simulink model "Eskf"  (R2025b)
settings: Solver=FixedStepDiscrete  StartTime=0.0  StopTime=100  FixedStep=Ts_10us  RelTol=1e-3
model workspace (MAT data in the model file):
  B_const = Simulink.Parameter
  B_const.Value = [1; 0; 0]
  B_const.Complexity = 'real'
  B_const.Dimensions = [3 1]
  B_const.DataType = 'auto'
  Param = Simulink.Parameter
  Param.Complexity = 'real'
  Param.Dimensions = [0 0]
  Param.DataType = 'auto'
  Ts_100us = Simulink.Parameter
  Ts_100us.Value = 0.0001
  Ts_100us.Complexity = 'real'
  Ts_100us.Dimensions = [1 1]
  Ts_100us.DataType = 'auto'
  Ts_10us = Simulink.Parameter
  Ts_10us.Value = 1e-05
  Ts_10us.Complexity = 'real'
  Ts_10us.Dimensions = [1 1]
  Ts_10us.DataType = 'auto'
  Ts_acc = Simulink.Parameter
  Ts_acc.Value = 0.0001
  Ts_acc.Complexity = 'real'
  Ts_acc.Dimensions = [1 1]
  Ts_acc.DataType = 'auto'
  Ts_eskf = Simulink.Parameter
  Ts_eskf.Value = 0.0001
  Ts_eskf.Complexity = 'real'
  Ts_eskf.Dimensions = [1 1]
  Ts_eskf.DataType = 'auto'
  Ts_gps = Simulink.Parameter
  Ts_gps.Value = 0.0001
  Ts_gps.Complexity = 'real'
  Ts_gps.Dimensions = [1 1]
  Ts_gps.DataType = 'auto'
  Ts_gyro = Simulink.Parameter
  Ts_gyro.Value = 0.0001
  Ts_gyro.Complexity = 'real'
  Ts_gyro.Dimensions = [1 1]
  Ts_gyro.DataType = 'auto'
  Ts_mag = Simulink.Parameter
  Ts_mag.Value = 0.0001
  Ts_mag.Complexity = 'real'
  Ts_mag.Dimensions = [1 1]
  Ts_mag.DataType = 'auto'
  acc_bias_static = Simulink.Parameter
  acc_bias_static.Value = [0.01; -0.01; 0.01]
  acc_bias_static.Complexity = 'real'
  acc_bias_static.Dimensions = [3 1]
  acc_bias_static.DataType = 'auto'
  g = Simulink.Parameter
  g.Value = [0; 0; 9.80665]
  g.Complexity = 'real'
  g.Dimensions = [3 1]
  g.DataType = 'auto'
  omega_bias_static = Simulink.Parameter
  omega_bias_static.Value = [0.01; -0.01; 0.01]
  omega_bias_static.Complexity = 'real'
  omega_bias_static.Dimensions = [3 1]
  omega_bias_static.DataType = 'auto'
  var_B_n = Simulink.Parameter
  var_B_n.Value = Simulink.data.Expression
  var_B_n.Value.ExpressionString = "0.001*[0.001;0.001;0.001]"
  var_B_n.Complexity = 'real'
  var_B_n.Dimensions = -1
  var_B_n.DataType = 'auto'
  var_a_n = Simulink.Parameter
  var_a_n.Value = Simulink.data.Expression
  var_a_n.Value.ExpressionString = "0.001"
  var_a_n.Complexity = 'real'
  var_a_n.Dimensions = -1
  var_a_n.DataType = 'auto'
  var_a_w = Simulink.Parameter
  var_a_w.Value = Simulink.data.Expression
  var_a_w.Value.ExpressionString = "0.001"
  var_a_w.Complexity = 'real'
  var_a_w.Dimensions = -1
  var_a_w.DataType = 'auto'
  var_pos_n = Simulink.Parameter
  var_pos_n.Value = Simulink.data.Expression
  var_pos_n.Value.ExpressionString = "0.001*[1;1;1]"
  var_pos_n.Complexity = 'real'
  var_pos_n.Dimensions = -1
  var_pos_n.DataType = 'auto'
  var_vel_n = Simulink.Parameter
  var_vel_n.Value = Simulink.data.Expression
  var_vel_n.Value.ExpressionString = "0.001*[0.1;0.1;0.1]"
  var_vel_n.Complexity = 'real'
  var_vel_n.Dimensions = -1
  var_vel_n.DataType = 'auto'
  var_w_n = Simulink.Parameter
  var_w_n.Value = Simulink.data.Expression
  var_w_n.Value.ExpressionString = "0.001"
  var_w_n.Complexity = 'real'
  var_w_n.Dimensions = -1
  var_w_n.DataType = 'auto'
  var_w_w = Simulink.Parameter
  var_w_w.Value = Simulink.data.Expression
  var_w_w.Value.ExpressionString = "0.001"
  var_w_w.Complexity = 'real'
  var_w_w.Dimensions = -1
  var_w_w.DataType = 'auto'
undefined symbols (not defined in the file): DiscIntNeverNeededParam
libraries: simulink x4
settings Model: Creator=unimage  LastModifiedBy=unimage
settings DebuggingCC: SignalInfNanChecking=error  CheckMatrixSingularityMsg=error

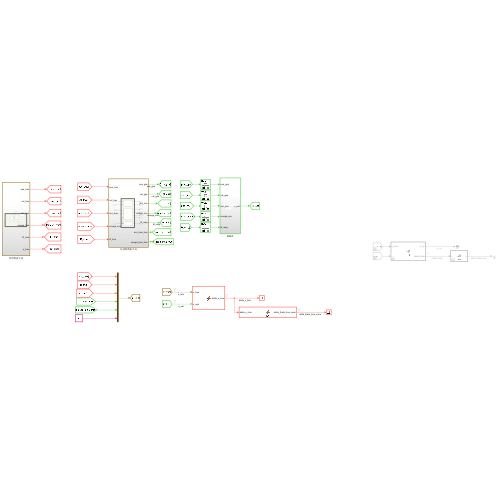
[thumbnail: Simulink's stored preview of the top-level diagram]
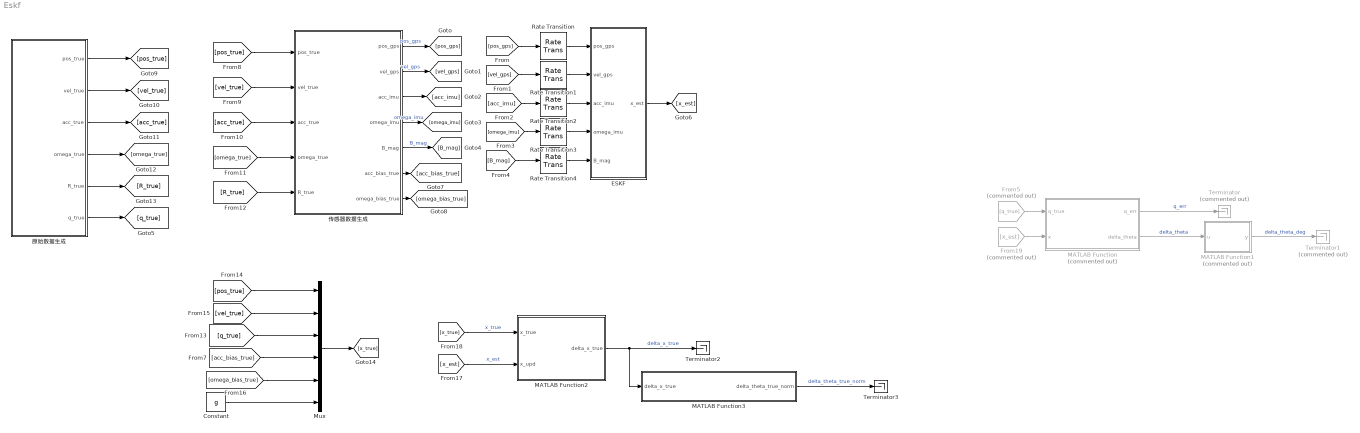
== system Eskf ==
  Constant : Constant  Value=g
  ESKF : Subsystem
  From19 : From  Commented=on  GotoTag=x_est
  From5 : From  Commented=on  GotoTag=q_true
  MATLAB Function : MATLAB Function  Commented=on  TreatAsAtomicUnit=on
  MATLAB Function1 : MATLAB Function  Commented=on  TreatAsAtomicUnit=on
  MATLAB Function2 : MATLAB Function  TreatAsAtomicUnit=on
  MATLAB Function3 : MATLAB Function  TreatAsAtomicUnit=on
  Mux : Mux  Inputs=6
  Rate Transition{,1..4} (5 alike) : RateTransition  OutPortSampleTime=Ts_eskf
  Terminator : Terminator  Commented=on
  Terminator1 : Terminator  Commented=on
  Terminator2 : Terminator
  Terminator3 : Terminator
  传感器数据生成 : Subsystem
  原始数据生成 : Subsystem
  wires:
  传感器数据生成/1(pos_gps) -> [pos_gps]  "pos_gps"
  传感器数据生成/2(vel_gps) -> [vel_gps]  "vel_gps"
  传感器数据生成/3(acc_imu) -> [acc_imu]
  传感器数据生成/4(omega_imu) -> [omega_imu]  "omega_imu"
  传感器数据生成/5(B_mag) -> [B_mag]  "B_mag"
  [pos_gps] -> Rate Transition/1
  [vel_gps] -> Rate Transition1/1
  [acc_imu] -> Rate Transition2/1
  [omega_imu] -> Rate Transition3/1
  [B_mag] -> Rate Transition4/1
  Rate Transition/1 -> ESKF/1(pos_gps)
  Rate Transition1/1 -> ESKF/2(vel_gps)
  Rate Transition2/1 -> ESKF/3(acc_imu)
  Rate Transition3/1 -> ESKF/4(omega_imu)
  Rate Transition4/1 -> ESKF/5(B_mag)
  原始数据生成/6(q_true) -> [q_true]
  ESKF/1(x_est) -> [x_est]
  From5/1 -> MATLAB Function/1(q_true)
  From19/1 -> MATLAB Function/2(x)
  MATLAB Function/1(q_err) -> Terminator/1  "q_err"
  MATLAB Function/2(delta_theta) -> MATLAB Function1/1(u)  "delta_theta"
  MATLAB Function1/1(y) -> Terminator1/1  "delta_theta_deg"
  传感器数据生成/6(acc_bias_true) -> [acc_bias_true]
  传感器数据生成/7(omega_bias_true) -> [omega_bias_true]
  原始数据生成/1(pos_true) -> [pos_true]
  原始数据生成/3(acc_true) -> [acc_true]
  原始数据生成/2(vel_true) -> [vel_true]
  原始数据生成/4(omega_true) -> [omega_true]
  原始数据生成/5(R_true) -> [R_true]
  [pos_true] -> 传感器数据生成/1(pos_true)
  [vel_true] -> 传感器数据生成/2(vel_true)
  [acc_true] -> 传感器数据生成/3(acc_true)
  [omega_true] -> 传感器数据生成/4(omega_true)
  [R_true] -> 传感器数据生成/5(R_true)
  [acc_bias_true] -> Mux/4
  [q_true] -> Mux/3
  [pos_true] -> Mux/1
  [vel_true] -> Mux/2
  [omega_bias_true] -> Mux/5
  Constant/1 -> Mux/6
  Mux/1 -> [x_true]
  [x_true] -> MATLAB Function2/1(x_true)  "x_true"
  [x_est] -> MATLAB Function2/2(x_upd)  "x_est"
  MATLAB Function2/1(delta_x_true) -> MATLAB Function3/1(delta_x_true), Terminator2/1  "delta_x_true"
  MATLAB Function3/1(delta_theta_true_norm) -> Terminator3/1  "delta_theta_true_norm"

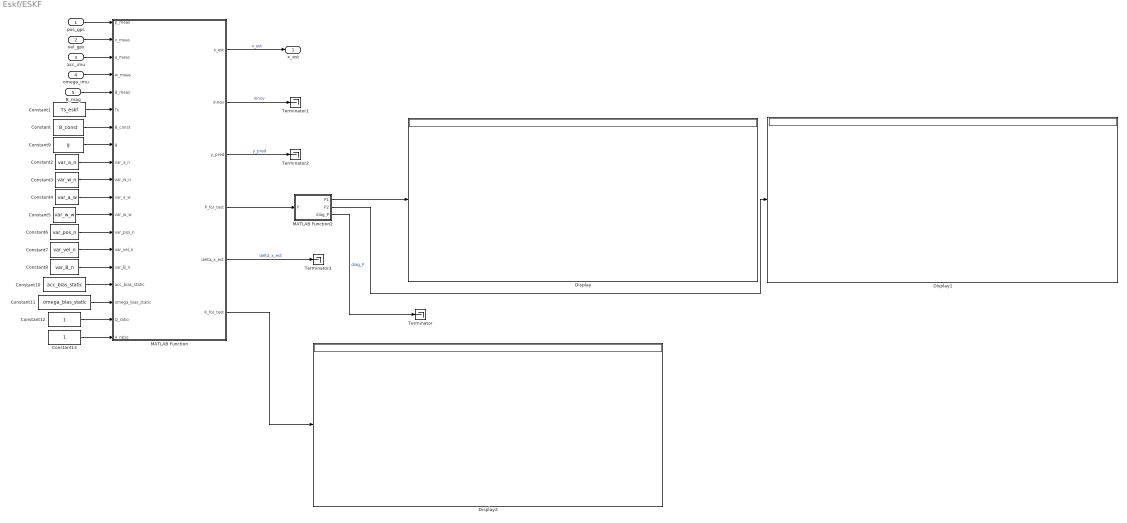
== system Eskf/ESKF ==
  pos_gps : Inport
  vel_gps : Inport  Port=2
  acc_imu : Inport  Port=3
  omega_imu : Inport  Port=4
  B_mag : Inport  Port=5
  Constant : Constant  Value=B_const
  Constant1 : Constant  Value=Ts_eskf
  Constant10 : Constant  Value=acc_bias_static
  Constant11 : Constant  Value=omega_bias_static
  Constant12 : Constant
  Constant13 : Constant
  Constant2 : Constant  Value=var_a_n
  Constant3 : Constant  Value=var_w_n
  Constant4 : Constant  Value=var_a_w
  Constant5 : Constant  Value=var_w_w
  Constant6 : Constant  Value=var_pos_n
  Constant7 : Constant  Value=var_vel_n
  Constant8 : Constant  Value=var_B_n
  Constant9 : Constant  Value=g
  Display : Display
      settings: Format=bank
  Display1 : Display
      settings: Format=bank
  Display2 : Display
      settings: Format=bank
  MATLAB Function : MATLAB Function  TreatAsAtomicUnit=on
  MATLAB Function2 : MATLAB Function  TreatAsAtomicUnit=on
  Terminator{,1..3} (4 alike) : Terminator
  x_est : Outport
  wires:
  pos_gps/1 -> MATLAB Function/1(p_meas)
  vel_gps/1 -> MATLAB Function/2(v_meas)
  acc_imu/1 -> MATLAB Function/3(a_meas)
  omega_imu/1 -> MATLAB Function/4(w_meas)
  B_mag/1 -> MATLAB Function/5(B_meas)
  Constant1/1 -> MATLAB Function/6(Ts)
  Constant/1 -> MATLAB Function/7(B_const)
  Constant2/1 -> MATLAB Function/9(var_a_n)
  Constant3/1 -> MATLAB Function/10(var_w_n)
  Constant4/1 -> MATLAB Function/11(var_a_w)
  Constant5/1 -> MATLAB Function/12(var_w_w)
  MATLAB Function/1(x_est) -> x_est/1  "x_est"
  MATLAB Function/2(innov) -> Terminator1/1  "innov"
  Constant6/1 -> MATLAB Function/13(var_pos_n)
  Constant7/1 -> MATLAB Function/14(var_vel_n)
  Constant8/1 -> MATLAB Function/15(var_B_n)
  MATLAB Function/3(y_pred) -> Terminator2/1  "y_pred"
  MATLAB Function/4(P_for_test) -> MATLAB Function2/1(P)
  MATLAB Function2/1(P1) -> Display/1
  MATLAB Function2/2(P2) -> Display1/1
  MATLAB Function2/3(diag_P) -> Terminator/1  "diag_P"
  MATLAB Function/5(delta_x_est) -> Terminator3/1  "delta_x_est"
  Constant9/1 -> MATLAB Function/8(g)
  Constant10/1 -> MATLAB Function/16(acc_bias_static)
  Constant11/1 -> MATLAB Function/17(omega_bias_static)
  Constant12/1 -> MATLAB Function/18(Q_ratio)
  Constant13/1 -> MATLAB Function/19(V_ratio)
  MATLAB Function/6(K_for_test) -> Display2/1

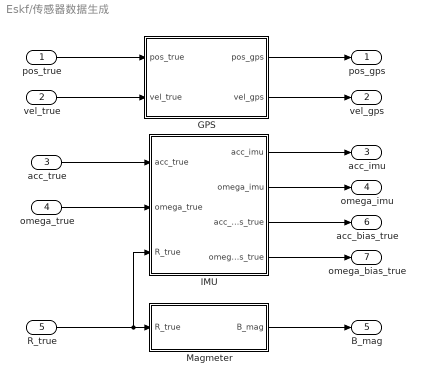
== system Eskf/传感器数据生成 ==
  pos_true : Inport
  vel_true : Inport  Port=2
  acc_true : Inport  Port=3
  omega_true : Inport  Port=4
  R_true : Inport  Port=5
  GPS : Subsystem
  IMU : Subsystem
  Magmeter : Subsystem
  pos_gps : Outport
  vel_gps : Outport  Port=2
  acc_imu : Outport  Port=3
  omega_imu : Outport  Port=4
  B_mag : Outport  Port=5
  acc_bias_true : Outport  Port=6
  omega_bias_true : Outport  Port=7
  wires:
  vel_true/1 -> GPS/2(vel_true)
  R_true/1 -> IMU/3(R_true), Magmeter/1(R_true)
  omega_true/1 -> IMU/2(omega_true)
  IMU/2(omega_imu) -> omega_imu/1
  IMU/1(acc_imu) -> acc_imu/1
  Magmeter/1(B_mag) -> B_mag/1
  acc_true/1 -> IMU/1(acc_true)
  pos_true/1 -> GPS/1(pos_true)
  GPS/1(pos_gps) -> pos_gps/1
  GPS/2(vel_gps) -> vel_gps/1
  IMU/3(acc_bias_true) -> acc_bias_true/1
  IMU/4(omega_bias_true) -> omega_bias_true/1

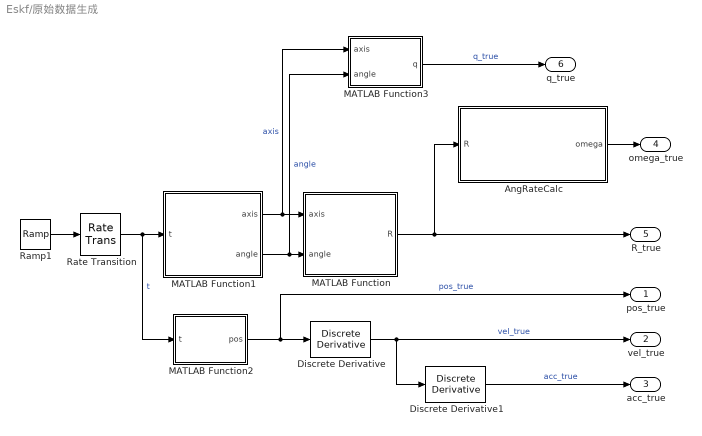
== system Eskf/原始数据生成 ==
  AngRateCalc : Subsystem
  Discrete Derivative : simulink/Discrete/Discrete Derivative  gainval=1.0  ICPrevScaledInput=0.0  OutMin=[]  OutMax=[]  OutDataType=fixdt(1, 16)  OutScaling=2^-10  DoSatur=off
  Discrete Derivative1 : simulink/Discrete/Discrete Derivative  gainval=1.0  ICPrevScaledInput=0.0  OutMin=[]  OutMax=[]  OutDataType=fixdt(1, 16)  OutScaling=2^-10  DoSatur=off
  MATLAB Function : MATLAB Function  TreatAsAtomicUnit=on
  MATLAB Function1 : MATLAB Function  TreatAsAtomicUnit=on
  MATLAB Function2 : MATLAB Function  TreatAsAtomicUnit=on
  MATLAB Function3 : MATLAB Function  TreatAsAtomicUnit=on
  Ramp1 : simulink/Sources/Ramp  slope=1  start=0  InitialOutput=0
  Rate Transition : RateTransition  OutPortSampleTime=Ts_10us
  pos_true : Outport
  vel_true : Outport  Port=2
  acc_true : Outport  Port=3
  omega_true : Outport  Port=4
  R_true : Outport  Port=5
  q_true : Outport  Port=6
  wires:
  MATLAB Function1/1(axis) -> MATLAB Function3/1(axis), MATLAB Function/1(axis)  "axis"
  MATLAB Function1/2(angle) -> MATLAB Function3/2(angle), MATLAB Function/2(angle)  "angle"
  MATLAB Function2/1(pos) -> pos_true/1, Discrete Derivative/1  "pos_true"
  Ramp1/1 -> Rate Transition/1
  Rate Transition/1 -> MATLAB Function2/1(t), MATLAB Function1/1(t)  "t"
  Discrete Derivative/1 -> vel_true/1, Discrete Derivative1/1  "vel_true"
  Discrete Derivative1/1 -> acc_true/1  "acc_true"
  AngRateCalc/1(omega) -> omega_true/1
  MATLAB Function/1(R) -> AngRateCalc/1(R), R_true/1
  MATLAB Function3/1(q) -> q_true/1  "q_true"

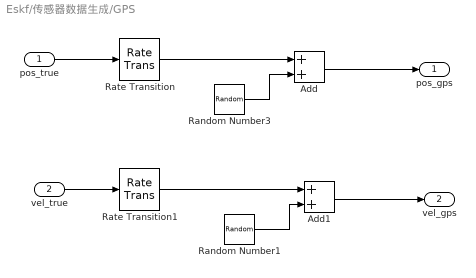
== system Eskf/传感器数据生成/GPS ==
  pos_true : Inport
  vel_true : Inport  Port=2
  Add : Sum
  Add1 : Sum
  Random Number1 : RandomNumber  Mean=[0 0 0]  Variance=var_vel_n  Seed=[0 1 2]  SampleTime=Ts_gps
  Random Number3 : RandomNumber  Mean=[0 0 0]  Variance=var_pos_n  Seed=[0 1 2]  SampleTime=Ts_gps
  Rate Transition : RateTransition  OutPortSampleTime=Ts_gps
  Rate Transition1 : RateTransition  OutPortSampleTime=Ts_gps
  pos_gps : Outport
  vel_gps : Outport  Port=2
  wires:
  pos_true/1 -> Rate Transition/1
  Random Number3/1 -> Add/2
  Add/1 -> pos_gps/1
  Random Number1/1 -> Add1/2
  vel_true/1 -> Rate Transition1/1
  Add1/1 -> vel_gps/1
  Rate Transition/1 -> Add/1
  Rate Transition1/1 -> Add1/1

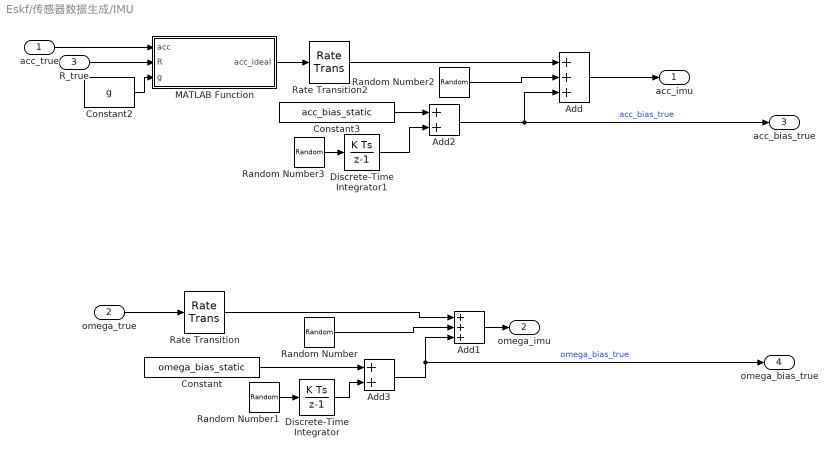
== system Eskf/传感器数据生成/IMU ==
  acc_true : Inport
  omega_true : Inport  Port=2
  R_true : Inport  Port=3
  Add : Sum  Inputs=+++
  Add1 : Sum  Inputs=+++
  Add2 : Sum
  Add3 : Sum
  Constant : Constant  Value=omega_bias_static
  Constant2 : Constant  Value=g
  Constant3 : Constant  Value=acc_bias_static
  Discrete-Time Integrator : DiscreteIntegrator  SampleTime=-1  ICPrevOutput=DiscIntNeverNeededParam  ICPrevScaledInput=DiscIntNeverNeededParam
  Discrete-Time Integrator1 : DiscreteIntegrator  SampleTime=-1  ICPrevOutput=DiscIntNeverNeededParam  ICPrevScaledInput=DiscIntNeverNeededParam
  MATLAB Function : MATLAB Function  TreatAsAtomicUnit=on
  Random Number : RandomNumber  Mean=[0 0 0]  Variance=var_w_n*ones(3,1)  Seed=[0 1 2]  SampleTime=Ts_gyro
  Random Number1 : RandomNumber  Mean=[0 0 0]  Variance=var_w_w*ones(3,1)  Seed=[3 4 5]  SampleTime=Ts_gyro
  Random Number2 : RandomNumber  Mean=[0 0 0]  Variance=var_a_n*ones(3,1)  Seed=[9 10 11]  SampleTime=Ts_acc
  Random Number3 : RandomNumber  Mean=[0 0 0]  Variance=var_a_w*ones(3,1)  Seed=[6 7 8]  SampleTime=Ts_acc
  Rate Transition : RateTransition  OutPortSampleTime=Ts_gyro
  Rate Transition2 : RateTransition  OutPortSampleTime=Ts_acc
  acc_imu : Outport
  omega_imu : Outport  Port=2
  acc_bias_true : Outport  Port=3
  omega_bias_true : Outport  Port=4
  wires:
  acc_true/1 -> MATLAB Function/1(acc)
  Add/1 -> acc_imu/1
  Random Number2/1 -> Add/2
  Constant3/1 -> Add2/1
  Add1/1 -> omega_imu/1
  omega_true/1 -> Rate Transition/1
  Random Number/1 -> Add1/2
  Random Number1/1 -> Discrete-Time Integrator/1
  Discrete-Time Integrator/1 -> Add3/2
  Constant/1 -> Add3/1
  Rate Transition/1 -> Add1/1
  Rate Transition2/1 -> Add/1
  MATLAB Function/1(acc_ideal) -> Rate Transition2/1
  R_true/1 -> MATLAB Function/2(R)
  Constant2/1 -> MATLAB Function/3(g)
  Random Number3/1 -> Discrete-Time Integrator1/1
  Discrete-Time Integrator1/1 -> Add2/2
  Add2/1 -> acc_bias_true/1, Add/3  "acc_bias_true"
  Add3/1 -> omega_bias_true/1, Add1/3  "omega_bias_true"

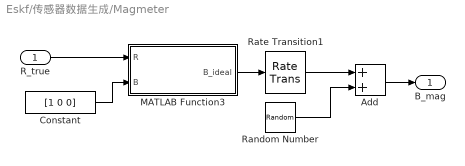
== system Eskf/传感器数据生成/Magmeter ==
  R_true : Inport
  Add : Sum
  Constant : Constant  Value=[1 0 0]
  MATLAB Function3 : MATLAB Function  TreatAsAtomicUnit=on
  Random Number : RandomNumber  Mean=[0 0 0]  Variance=var_B_n  Seed=[13 14 15]  SampleTime=Ts_mag
  Rate Transition1 : RateTransition  OutPortSampleTime=Ts_mag
  B_mag : Outport
  wires:
  MATLAB Function3/1(B_ideal) -> Rate Transition1/1
  Add/1 -> B_mag/1
  Random Number/1 -> Add/2
  Rate Transition1/1 -> Add/1
  R_true/1 -> MATLAB Function3/1(R)
  Constant/1 -> MATLAB Function3/2(B)

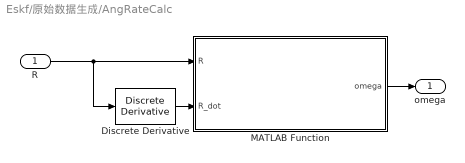
== system Eskf/原始数据生成/AngRateCalc ==
  R : Inport
  Discrete Derivative : simulink/Discrete/Discrete Derivative  gainval=1.0  ICPrevScaledInput=0.0  OutMin=[]  OutMax=[]  OutDataType=fixdt(1, 16)  OutScaling=2^-10  DoSatur=off
  MATLAB Function : MATLAB Function  TreatAsAtomicUnit=on
  omega : Outport
  wires:
  R/1 -> MATLAB Function/1(R), Discrete Derivative/1
  Discrete Derivative/1 -> MATLAB Function/2(R_dot)
  MATLAB Function/1(omega) -> omega/1

== matlab function Eskf/MATLAB Function ==
  data: q_true input; q_err output; x input; delta_theta output
function [q_err,delta_theta] = fcn(q_true,x)

q_nom = x(7:10);                                %dv

q_err = q_product(q_inv(q_true),q_nom);         %dv

delta_theta = 2*asin(norm(q_err(2:4)));         %dv

end



function out = q_inv(q)                             %dv
    out = 1/(norm(q)^2)*[q(1);-q(2:4)];             %dv
end


function out = q_product(p,q)                                       %dv
    out = [         p(1)*q(1) - p(2:4)'*q(2:4);                     %dv
            p(1)*q(2:4) + q(1)*p(2:4) + cross(p(2:4),q(2:4));];     %dv
end

== matlab function Eskf/原始数据生成/MATLAB Function3 ==
  data: axis input; q output; angle input
function q = fcn(axis, angle)

q = [cos(angle/2);sin(angle/2)*axis];

end

== matlab function Eskf/ESKF/MATLAB Function2 ==
  data: P input; P1 output; P2 output; diag_P output
function [P1,P2,diag_P] = fcn(P)

P1 = P(1:18,1:9);
P2 = P(1:18,10:18);
diag_P = diag(P);

end

== matlab function Eskf/MATLAB Function1 ==
  data: u input; y output
function y = fcn(u)


y = u/pi*180;


end

== matlab function Eskf/MATLAB Function2 ==
  data: x_true input; delta_x_true output; x_upd input
function delta_x_true = fcn(x_true, x_upd)

delta_x_true = zeros(18,1);
delta_x_true(1:6) = x_true(1:6) - x_upd(1:6);
delta_x_true(10:18) = x_true(11:19) - x_upd(11:19);

q_true = x_true(7:10);
q_upd = x_upd(7:10);

delta_q = q_product(q_inv(q_upd),q_true);
if(norm(delta_q(2:4)) > 1e-5)
    delta_theta_norm = 2*asin(norm(delta_q(2:4)));
    delta_theta_direc = delta_q(2:4)/norm(delta_q(2:4));
    delta_x_true(7:9) = delta_theta_norm*delta_theta_direc;
else
    delta_x_true(7:9) = zeros(3,1);
end

end


function out = q_product(p,q)
    out = [         p(1)*q(1) - p(2:4)'*q(2:4);
            p(1)*q(2:4) + q(1)*p(2:4) + cross(p(2:4),q(2:4));];
end

function out = q_inv(in)
    out = [in(1);-in(2:4)];
    out = out/(norm(out)^2);
end

== matlab function Eskf/MATLAB Function3 ==
  data: delta_x_true input; delta_theta_true_norm output
function delta_theta_true_norm = fcn(delta_x_true)

delta_theta_true_norm = norm(delta_x_true(7:9));
delta_theta_true_norm = delta_theta_true_norm/pi*180;
end

== matlab function Eskf/原始数据生成/MATLAB Function1 ==
  data: t input size=[1 1]; axis output size=[3 1]; angle output size=[1 1]
function [axis,angle] = fcn(t)  %dv

axis = [sin(t);1;0;];              %dv
axis = axis/norm(axis);        %dv
angle = cos(t)-1;                   %dv
angle = mod(angle,2*pi);       %dv

end

== matlab function Eskf/原始数据生成/MATLAB Function ==
  data: axis input; R output; angle input
function R  = fcn(axis, angle)                      %dv

R = expm(angle*skew(axis));                         %dv

end


function out = skew(in)                             %dv
    out = [ 0,     -in(3),   in(2);                 %dv
           in(3),    0,     -in(1);                 %dv
          -in(2),   in(1),     0; ];                %dv
end                                                 %dv

== matlab function Eskf/原始数据生成/AngRateCalc/MATLAB Function ==
  data: R input; omega output; R_dot input
function omega = fcn(R, R_dot)          %dv

omega_skew = R\R_dot;                   %dv
omega = anti_skew(omega_skew);          %dv

end

function out = anti_skew(in)            %dv
    out = [in(3,2);                     %dv
           in(1,3);                     %dv
           in(2,1);];                   %dv
end

== matlab function Eskf/原始数据生成/MATLAB Function2 ==
  data: t input; pos output
function pos = fcn(t)               %dv

pos = [t^2;2*t^2;3*t^2];                      %dv


end

== matlab function Eskf/传感器数据生成/Magmeter/MATLAB Function3 ==
  data: R input; B_ideal output; B input
function B_ideal = fcn(R,B)             %dv

B_ideal = R\B;                 %dv

end

== matlab function Eskf/传感器数据生成/IMU/MATLAB Function ==
  data: acc input; acc_ideal output; R input; g input
function acc_ideal = fcn(acc,R,g)       %dv

acc_ideal = R\(acc-g);                  %dv

end                                     %dv

== matlab function Eskf/ESKF/MATLAB Function ==
  data: p_meas input; x_est output; v_meas input; a_meas input; w_meas input; B_meas input; Ts input; B_const input; g input; var_a_n input; var_w_n input; var_a_w input; var_w_w input; innov output; var_pos_n input; var_vel_n input; var_B_n input; y_pred output; P_for_test output; delta_x_est output; acc_bias_static input; omega_bias_static input; Q_ratio input; V_ratio input; K_for_test output
function [x_est,innov,y_pred,P_for_test,delta_x_est,K_for_test] = fcn(p_meas, v_meas, a_meas, w_meas, B_meas, Ts,B_const,g,var_a_n,var_w_n,var_a_w,var_w_w, var_pos_n, var_vel_n, var_B_n, acc_bias_static, omega_bias_static,Q_ratio,V_ratio)


persistent P;                               %dv
if(isempty(P))                              %dv
    P = 1*eye(18);                       %dv     %?初值具体如何设置
end

persistent x_nom;                           %dv
if(isempty(x_nom))                          %dv     %?初始值如何设置
    x_nom = zeros(19,1);                    %dv
    x_nom(1:3) = p_meas;                    %dv
    x_nom(4:6) = v_meas;                    %dv
    x_nom(7:10) = [1;0;0;0];                %dv
    x_nom(11:13) = acc_bias_static;         %dv
    x_nom(14:16) = omega_bias_static;       %dv
    x_nom(17:19) = g;                       %dv
end

persistent V;                               %dv 观测噪声协方差矩阵
if(isempty(V))                              %dv
    V = diag([var_pos_n;var_vel_n;var_B_n]);%dv
    V = V_ratio*V;
end                                         %dv




    
% 1.误差状态预测（省略）                      %dv


% 2.名义状态积分                             %dv
p_nom = x_nom(1:3);                         %dv
v_nom = x_nom(4:6);                         %dv
q_nom = x_nom(7:10);                        %dv
a_bias_nom = x_nom(11:13);                  %dv
w_bias_nom = x_nom(14:16);                  %dv
g_nom = x_nom(17:19);                       %dv
p_nom_pred = p_nom + v_nom*Ts + 1/2*Ts^2*(q_to_R(q_nom)*(a_meas - a_bias_nom) + g_nom);         %dv
v_nom_pred = v_nom + Ts*(q_to_R(q_nom)*(a_meas - a_bias_nom) + g_nom);                          %dv
q_nom_pred = expm(Ts/2*right_mat([0;w_meas - w_bias_nom]))*q_nom;                               %dv
a_bias_nom_pred = a_bias_nom;                                                                   %dv
w_bias_nom_pred = w_bias_nom;                                                                   %dv
g_nom_pred = g_nom;                                                                             %dv
x_nom_pred =[p_nom_pred;v_nom_pred;q_nom_pred;a_bias_nom_pred;w_bias_nom_pred;g_nom_pred];      %dv

% 3.残差计算                                                %dv
y_meas = [p_meas;v_meas;B_meas];                           %dv
y_pred = zeros(9,1);                                       %dv
y_pred(1:3) = p_nom_pred;                                  %dv
y_pred(4:6) = v_nom_pred;                                  %dv
y_pred(7:9) = (q_to_R(q_nom_pred))\B_const;                %dv
innov = y_meas - y_pred;                                   %dv


% 协方差矩阵预测
F_x = [eye(3),          Ts*eye(3),               zeros(3,3),                                    zeros(3,3),            zeros(3,3),     zeros(3,3);      %dv
       zeros(3,3),      eye(3),      -Ts*q_to_R(q_nom_pred)*skew(a_meas - a_bias_nom_pred), -Ts*q_to_R(q_nom_pred),    zeros(3,3),     Ts*eye(3);       %dv
       zeros(3,3),      zeros(3,3),    expm(-Ts*skew(w_meas - w_bias_nom_pred)),                 zeros(3,3),          -Ts*eye(3),      zeros(3,3);      %dv
       zeros(3,3),      zeros(3,3),              zeros(3,3),                                     eye(3),               zeros(3,3),     zeros(3,3);      %dv
       zeros(3,3),      zeros(3,3),              zeros(3,3),                                     zeros(3,3),           eye(3),         zeros(3,3);      %dv
       zeros(3,3),      zeros(3,3),              zeros(3,3),                                     zeros(3,3),           zeros(3,3),       eye(3);];      %dv
                                            %？遗留问题：协方差矩阵预测公式中，名义状态该用预测值还是当前值？

F_i = [zeros(3,3),     zeros(3,3),     zeros(3,3),     zeros(3,3);          %dv
       eye(3),         zeros(3,3),     zeros(3,3),     zeros(3,3);          %dv
       zeros(3,3),     eye(3),         zeros(3,3),     zeros(3,3);          %dv
       zeros(3,3),     zeros(3,3),     eye(3),         zeros(3,3);          %dv
       zeros(3,3),     zeros(3,3),     zeros(3,3),     eye(3);              %dv
       zeros(3,3),     zeros(3,3),     zeros(3,3),     zeros(3,3);];        %dv

Q_i = [Ts*var_a_n*eye(3),     zeros(3,3),               zeros(3,3),              zeros(3,3);                %dv   ？原文中有错误
       zeros(3,3),            Ts*var_w_n*eye(3),        zeros(3,3),              zeros(3,3);                %dv
       zeros(3,3),            zeros(3,3),               Ts^2*var_a_w*eye(3),     zeros(3,3);                %dv
       zeros(3,3),            zeros(3,3),               zeros(3,3),           Ts^2*var_w_w*eye(3);];        %dv
Q_i = Q_ratio*Q_i;

P_pred = F_x*P*F_x' + F_i*Q_i*F_i';                                                                         %dv

H = [eye(3),           zeros(3,3),       zeros(3,3),                   zeros(3,3),       zeros(3,3),       zeros(3,3);           %dv
     zeros(3,3),       eye(3),           zeros(3,3),                   zeros(3,3),       zeros(3,3),       zeros(3,3);           %dv
     zeros(3,3),       zeros(3,3),   skew(q_to_R(q_nom_pred)\B_const), zeros(3,3),       zeros(3,3),       zeros(3,3);           %dv
     ];          %dv

% 计算卡尔曼增益
K = (P_pred*H')/(H*P_pred*H' + V);                      %dv


% 误差状态修正                                           
delta_x_est = K*innov;                                    %dv


% 协方差矩阵修正                                         %dv
P = (eye(18)-K*H)*P_pred*(eye(18)-K*H)' + K*V*K';       %dv


% 叠加
x_nom(1:3) = x_nom_pred(1:3) + delta_x_est(1:3);          %dv
x_nom(4:6) = x_nom_pred(4:6) + delta_x_est(4:6);          %dv

delta_theta = delta_x_est(7:9);                                                       %dv
delta_theta_norm = norm(delta_theta);                                               %dv
if(delta_theta_norm > 1e-6)
    delta_theta_direc = delta_theta/norm(delta_theta);                                  %dv
    delta_q = [cos(delta_theta_norm/2);    sin(delta_theta_norm/2)*delta_theta_direc];  %dv
else
    delta_q = [1;0;0;0];
end
x_nom(7:10) = q_product(x_nom_pred(7:10),delta_q);                                  %dv
x_nom(7:10) = x_nom(7:10)/norm(x_nom(7:10));                                        %dv

x_nom(11:13) = x_nom_pred(11:13) + delta_x_est(10:12);                                %dv
x_nom(14:16) = x_nom_pred(14:16) + delta_x_est(13:15);                                %dv
x_nom(17:19) = x_nom_pred(17:19) + delta_x_est(16:18);                                %dv

G = [eye(6),                 zeros(6,3),                 zeros(6,9);
     zeros(3,6),    eye(3)-skew(1/2*delta_x_est(7:9)),   zeros(3,9);
     zeros(9,6),            zeros(9,3),                  eye(9);   ];

P = G*P*G';

x_est = x_nom;                                                                          %dv
P_for_test = P;                                                                     %dv
K_for_test = K;

end                                                                                 %dv



function out = q_product(p,q)
    out = [         p(1)*q(1) - p(2:4)'*q(2:4);
            p(1)*q(2:4) + q(1)*p(2:4) + cross(p(2:4),q(2:4));];
end

function out = right_mat(in)
    out = [in(1),   -in(2),   -in(3),   -in(4);
           in(2),    in(1),    in(4),   -in(3);
           in(3),   -in(4),    in(1),    in(2);
           in(4),    in(3),   -in(2),    in(1);];
end

function out = q_to_R(in)
    out = (in(1)^2 - in(2:4)'*in(2:4))*eye(3) + 2*in(2:4)*in(2:4)' + 2*in(1)*skew(in(2:4));
end


function out = skew(in)
    out = [ 0,     -in(3),   in(2);
           in(3),    0,     -in(1);
          -in(2),   in(1),     0; ];
end
